simulink model "tx_to_usrp"  (R2014b)
settings: Solver=FixedStepDiscrete  SolverMode=SingleTasking  StartTime=0.0  StopTime=5  FixedStep=1/2e6  MaxStep=1/(100*40e6)  RelTol=1e-3
PreLoadFcn:
  | Fsymbol              = .5e6;         % Symbol rate
  | D=8;  % decimation / interpolation
  | Bits_per_Symbol = 2;
  | Fbit  = Bits_per_Symbol*Fsymbol;
  | 
  | FFT_Size  = 64;
  | Cyclic        = 16;
  | Pilots         = 16;
  | Pilot_Level = 8;
  | Zero_Pad  = 3;
  | QAM_Level = 6;
  | 
  | OFDM_Frame =  FFT_Size+Cyclic;
  | Symbols_per_Frame = FFT_Size-Pilots-Zero_Pad;
  | 
  | Bits_per_Frame = Bits_per_Symbol*Symbols_per_Frame;
  | 
  | F_nco = Fsymbol*D*OFDM_Frame/(Symbols_per_Frame);
  | nco_nominal=2/D;
  | 
  | 
  | Fdelay = 8;  % rrc filter delay
  | Alpha = .25;  % excess BW
  | %rrc_coef=rcosine(1,D,'fir/sqrt',Alpha,Fdelay);
  | %rrc_coef=rrc_coef/sum(rrc_coef);
  | 
  | DPS=fdesign.pulseshaping(D,'Square Root Raised Cosine','Nsym,Beta',2*Fdelay,Alpha);
  | Hd=design(DPS);
  | rrc_coef=Hd.Numerator;
  | % force DC gain to unity.
  | rrc_coef=rrc_coef/sum(rrc_coef);
  | 
  | % coefficents for Farrow filter
  | b3 = [1/6 -1/2  1/2 -1/6];
  | b2 = [1/2 -1    1/2  0];
  | b1 = [1/3  1/2 -1    1/6];
  | b0 = [0    1    0    0];
StartFcn:
  | tic
StopFcn:
  | trun=toc
undefined symbols (not defined in the file or in its folder): dfilt, j
libraries: simulink x10, dspsigops x4, dspobslib x3, commchan3 x2, commrandsrc2 x1, dspxfrm3 x1, commdigbbndam3 x1, commsdrhw_v2 x1
Description:
  | Pilot Driven OFDM  Synchronization
settings Model: Creator=Dick Benson  LastModifiedBy=lubo
settings Model: ModifiedHistory=|
  | 12/8/07  D&C
  | 12/03/08  Added BER, tuned control loops, enhanced channel model.
settings DataIOCC: SignalLoggingSaveFormat=ModelDataLogs  SaveOutput=off  SignalLogging=off  SaveTime=off  SignalLoggingName=sigsOut
settings OptimizationCC: BlockReduction=off  BooleanDataType=off  ExpressionDepthLimit=2147483647  InitFltsAndDblsToZero=on
settings DebuggingCC: SaveWithParameterizedLinksMsg=none  UnderspecifiedInitializationDetection=Classic  MergeDetectMultiDrivingBlocksExec=none  SignalResolutionControl=TryResolveAllWithWarning  SolverPrmCheckMsg=none  InheritedTsInSrcMsg=none  MultiTaskDSMMsg=warning  MultiTaskCondExecSysMsg=none  ParameterPrecisionLossMsg=none  FcnCallInpInsideContextMsg=UseLocalSettings  StateNameClashWarn=warning
settings HardwareCC: TargetUnknown=on
settings SFSimCC: SimParseCustomCode=off
settings RTWCC: IncludeERTFirstTime=on
settings GRTTargetCC: TargetFcnLib=ansi_tfl_tmw.mat  CombineOutputUpdateFcns=off  GRTInterface=on

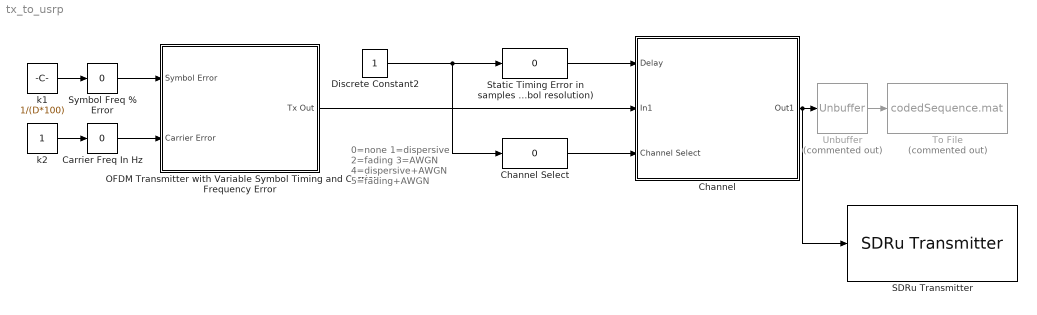
== system tx_to_usrp ==
  note: 0=none
      | 1=dispersive
      | 2=fading
      | 3=AWGN
      | 4=dispersive+AWGN
      | 5=fading+AWGN
  Carrier Freq In Hz : simulink/Math Operations/Slider Gain  low=-1000  gain=0  high=1000
  Channel : Subsystem
  Channel Select : simulink/Math Operations/Slider Gain  low=0  gain=0  high=5
  Discrete Constant2 : Constant  OutDataTypeStr=Inherit: Inherit via back propagation
  OFDM Transmitter with Variable Symbol Timing and Carrier Frequency Error : Subsystem
  SDRu Transmitter : commsdrhw_v2/SDRu Transmitter  rxtx=tx  platform=N200/N210/USRP2  USRP2_IP='192.168.10.2'  USRP_IP_X300='192.168.10.2'  USRP_IP_X310='192.168.10.2'  USRP_serialNumB200=''  USRP_serialNumB210=''  centerFrequency=8e6  centerFrequencySrc=Dialog  loOffset=0  loOffsetSrc=Dialog  masterClkRateB200=32e6  masterClkRateB210=32e6  masterClkRateX300=200e6  masterClkRateX310=200e6  masterClkRateParam=100e6  gain=8  gainSrc=Dialog  decimInterp=100  decimInterpSrc=Dialog  USRP2_IP_NUM=[49 57 50 46 49 54 56 46 49 48 46 50]  frameLength=362  outputDatatype=int16  overrunUnderrunPort=off  sampleTime=1  dboardInfo=|  HOST_DATA_PORT=30000  HOST_CONTROL_PORT=30001  USRP2_DATA_PORT=32769  USRP2_CONTROL_PORT=32768  bufferMode=Continuous streaming  EnableBurstMode=off  NumFramesInBurst=100  USRP_ID='192.168.10.2'
      | dbid: 0
      |           dbName: 'no db found'
      |          freqMin: 0
      |          freqMax: 0
      |          gainMin: 0
      |          gainMax: 0
      |     gainStepSize: 0
  Static Timing Error in samples (1/8 symbol resolution) : simulink/Math Operations/Slider Gain  low=-40  gain=0  high=40
  "Symbol Freq % Error " : simulink/Math Operations/Slider Gain  low=-0.5  gain=0  high=0.5
  To File : ToFile  Commented=on  Filename=codedSequence.mat  SaveFormat=Timeseries
  Unbuffer : Unbuffer  Commented=on  SampleBasedProcessing=Same as frame based
  k1 : Constant  Value=1/(D*100)
  k2 : Constant
  wires:
  k1/1 -> "Symbol Freq % Error "/1
  "Symbol Freq % Error "/1 -> OFDM Transmitter with Variable Symbol Timing and Carrier Frequency Error/1(Symbol Error)
  Carrier Freq In Hz/1 -> OFDM Transmitter with Variable Symbol Timing and Carrier Frequency Error/2(Carrier Error)
  k2/1 -> Carrier Freq In Hz/1
  OFDM Transmitter with Variable Symbol Timing and Carrier Frequency Error/1(Tx Out) -> Channel/2(In1)
  Discrete Constant2/1 -> Static Timing Error in samples (1/8 symbol resolution)/1, Channel Select/1
  Static Timing Error in samples (1/8 symbol resolution)/1 -> Channel/1(Delay)
  Channel Select/1 -> Channel/3(Channel Select)
  Channel/1(Out1) -> SDRu Transmitter/1, Unbuffer/1
  Unbuffer/1 -> To File/1

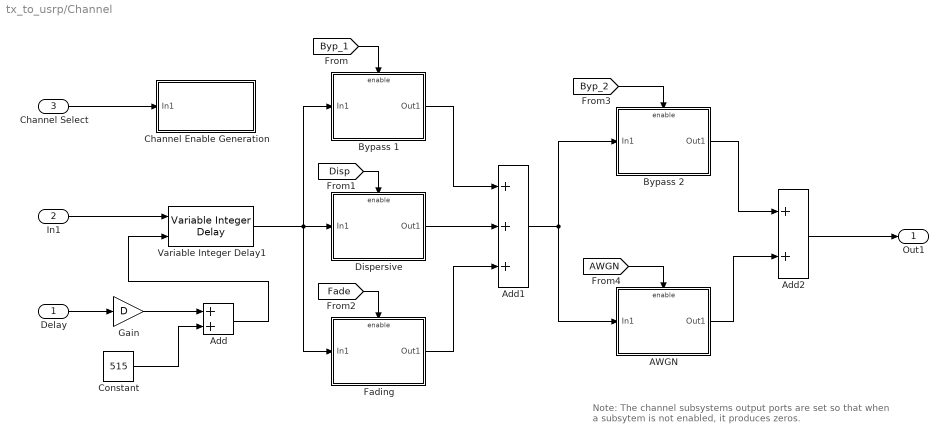
== system tx_to_usrp/Channel ==
  note: Note: The channel subsystems output ports are set so that
      | when a subsytem is not enabled, it produces zeros.
  Delay : Inport
  In1 : Inport  Port=2
  Channel Select : Inport  Port=3
  AWGN : Subsystem  TreatAsAtomicUnit=on
  Add : Sum
  Add1 : Sum  Inputs=+++
  Add2 : Sum
  Bypass 1 : Subsystem  TreatAsAtomicUnit=on
  Bypass 2 : Subsystem  TreatAsAtomicUnit=on
  Channel Enable Generation : Subsystem
  Constant : Constant  Value=515
  Dispersive : Subsystem  TreatAsAtomicUnit=on
  Fading : Subsystem  TreatAsAtomicUnit=on
  Gain : Gain  Gain=D
  Variable Integer Delay1 : dspobslib/Variable Integer Delay  dmax=2*516  InputProcessing=Columns as channels (frame based)  ic=0  noDFT=off
  Out1 : Outport
  wires:
  Delay/1 -> Gain/1
  Constant/1 -> Add/2
  Gain/1 -> Add/1
  Dispersive/1(Out1) -> Add1/2
  Bypass 1/1(Out1) -> Add1/1
  Fading/1(Out1) -> Add1/3
  Add1/1 -> AWGN/1(In1), Bypass 2/1(In1)
  Bypass 2/1(Out1) -> Add2/1
  AWGN/1(Out1) -> Add2/2
  Add2/1 -> Out1/1
  Channel Select/1 -> Channel Enable Generation/1(In1)
  [Byp_1] -> Bypass 1/Enable
  [Disp] -> Dispersive/Enable
  [Fade] -> Fading/Enable
  [Byp_2] -> Bypass 2/Enable
  [AWGN] -> AWGN/Enable
  Variable Integer Delay1/1 -> Dispersive/1(In1), Bypass 1/1(In1), Fading/1(In1)
  In1/1 -> Variable Integer Delay1/1
  Add/1 -> Variable Integer Delay1/2

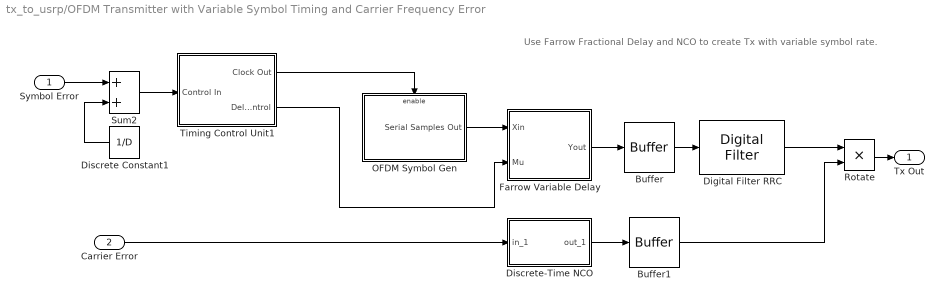
== system tx_to_usrp/OFDM Transmitter with Variable Symbol Timing and Carrier Frequency Error ==
  note: Use Farrow Fractional Delay and NCO to create Tx with variable symbol rate.
  Symbol Error : Inport
  Carrier Error : Inport  Port=2
  Buffer : Buffer  N=OFDM_Frame*D  TreatMby1Signals=One channel
  Buffer1 : Buffer  N=OFDM_Frame*D  TreatMby1Signals=One channel
  "Digital Filter RRC " : dspobslib/Digital Filter  TypePopup=FIR (all zeros)  IIRFiltStruct=Direct form II transposed  AllPoleFiltStruct=Direct form  FIRFiltStruct=Direct form  CoeffSource=Specify via dialog  NumCoeffs=rrc_coef  DenCoeffs=[1 0.1]  BiQuadCoeffs=[1 0.3 0.4 1 0.1 0.2]  LatticeCoeffs=[0.2 0.4]  denIgnore=on  FiltPerSampPopup=One filter per frame  IC=0  ICnum=0  ICden=0  roundingMode=Floor  overflowMode=off  ScaleValues=1  scaleValueFracLength=14  stageInFracLength=15  stageOutFracLength=15  FilterSource=Specify via dialog  dfiltObjectName=dfilt.dffir([1 2 1])  InputProcessing=Columns as channels (frame based)
  Discrete Constant1 : Constant  Value=1/D  OutDataTypeStr=Inherit: Inherit via back propagation
  Discrete-Time NCO : Subsystem  mask{Ac=1, Fc=0, Kc=1, Ph=0, ts=1/F_nco}
      mask prompts: Ac "Output amplitude:"; Fc "Oscillation frequency (Hz):"; Kc "Input sensitivity:"; Ph "Initial phase (rad):"; ts "Sample time:"
      mask init:
      | if ((length(Ac)~=1) | (length(Fc)~=1) | (length(Kc)~=1) | (length(Ph)~=1) | (length(ts)~=1) |(length(Ph)~=1))error('Mask parameters must be scalar values.');end;
      | pi2=2*pi;
      mask Display: disp('Discrete-Time\nNCO (rab)')
  Farrow Variable Delay : Subsystem
  OFDM Symbol Gen : Subsystem
  Rotate : Product  RndMeth=Zero
  Sum2 : Sum  SaturateOnIntegerOverflow=on  InputSameDT=on  OutDataTypeStr=Inherit: Same as first input
  Timing Control Unit1 : Subsystem
  Tx Out : Outport
  wires:
  Rotate/1 -> Tx Out/1
  Symbol Error/1 -> Sum2/1
  Farrow Variable Delay/1(Yout) -> Buffer/1
  Buffer/1 -> "Digital Filter RRC "/1
  "Digital Filter RRC "/1 -> Rotate/1
  Discrete-Time NCO/1(out_1) -> Buffer1/1
  Carrier Error/1 -> Discrete-Time NCO/1(in_1)
  Buffer1/1 -> Rotate/2
  Sum2/1 -> Timing Control Unit1/1(Control In)
  Timing Control Unit1/2(Delay Control) -> Farrow Variable Delay/2(Mu)
  Timing Control Unit1/1(Clock Out) -> OFDM Symbol Gen/Enable
  Discrete Constant1/1 -> Sum2/2
  OFDM Symbol Gen/1(Serial Samples Out) -> Farrow Variable Delay/1(Xin)

== system tx_to_usrp/Channel/AWGN ==
  In1 : Inport
  Enable : EnablePort
  AWGN Channel1 : commchan3/AWGN Channel  InputProcessing=Columns as channels (frame based)  seed=15  noiseMode="Signal to noise ratio  (SNR)"  EbNodB=10  EsNodB=10  SNRdB=15  bitsPerSym=1  Ps=1  Tsym=1  variance=1
  Out1 : Outport  OutputWhenDisabled=reset  InitialOutput=0+j*eps
  wires:
  In1/1 -> AWGN Channel1/1
  AWGN Channel1/1 -> Out1/1

== system tx_to_usrp/Channel/Bypass 1 ==
  In1 : Inport
  Enable : EnablePort
  Out1 : Outport  OutputWhenDisabled=reset  InitialOutput=0+j*eps
  wires:
  In1/1 -> Out1/1

== system tx_to_usrp/Channel/Bypass 2 ==
  In1 : Inport
  Enable : EnablePort
  Out1 : Outport  OutputWhenDisabled=reset  InitialOutput=0+j*eps
  wires:
  In1/1 -> Out1/1

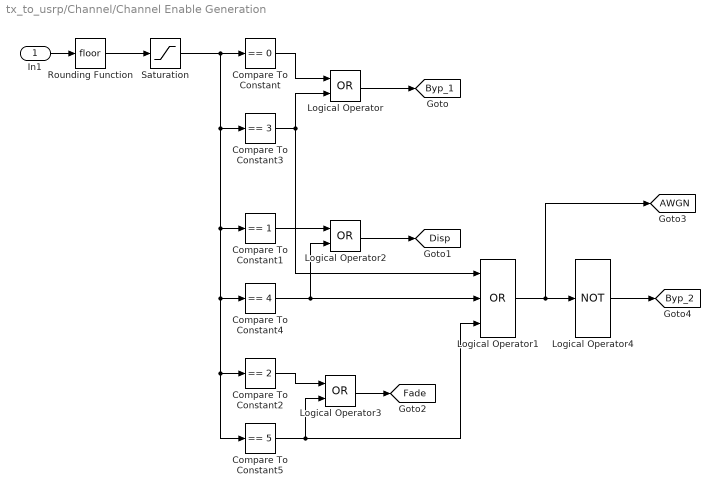
== system tx_to_usrp/Channel/Channel Enable Generation ==
  In1 : Inport
  Compare To Constant : simulink/Logic and Bit Operations/Compare To Constant  relop===  const=0  OutDataTypeStr=boolean  ZeroCross=off
  Compare To Constant1 : simulink/Logic and Bit Operations/Compare To Constant  relop===  const=1  OutDataTypeStr=boolean  ZeroCross=off
  Compare To Constant2 : simulink/Logic and Bit Operations/Compare To Constant  relop===  const=2  OutDataTypeStr=boolean  ZeroCross=off
  Compare To Constant3 : simulink/Logic and Bit Operations/Compare To Constant  relop===  const=3  OutDataTypeStr=boolean  ZeroCross=off
  Compare To Constant4 : simulink/Logic and Bit Operations/Compare To Constant  relop===  const=4  OutDataTypeStr=boolean  ZeroCross=off
  Compare To Constant5 : simulink/Logic and Bit Operations/Compare To Constant  relop===  const=5  OutDataTypeStr=boolean  ZeroCross=off
  Logical Operator : Logic  Operator=OR  AllPortsSameDT=off  OutDataTypeStr=boolean
  Logical Operator1 : Logic  Operator=OR  Inputs=3  AllPortsSameDT=off  OutDataTypeStr=boolean
  Logical Operator2 : Logic  Operator=OR  AllPortsSameDT=off  OutDataTypeStr=boolean
  Logical Operator3 : Logic  Operator=OR  AllPortsSameDT=off  OutDataTypeStr=boolean
  Logical Operator4 : Logic  Operator=NOT  Inputs=3  AllPortsSameDT=off  OutDataTypeStr=boolean
  Rounding Function : Rounding
  Saturation : Saturate  UpperLimit=5  LowerLimit=0  LinearizeAsGain=off
  tag scope: AWGN=global, Byp_1=global, Byp_2=global, Disp=global, Fade=global
  wires:
  In1/1 -> Rounding Function/1
  Compare To Constant/1 -> Logical Operator/1
  Compare To Constant3/1 -> Logical Operator/2, Logical Operator1/1
  Logical Operator/1 -> [Byp_1]
  Compare To Constant4/1 -> Logical Operator1/2, Logical Operator2/2
  Compare To Constant5/1 -> Logical Operator1/3, Logical Operator3/2
  Compare To Constant1/1 -> Logical Operator2/1
  Logical Operator2/1 -> [Disp]
  Compare To Constant2/1 -> Logical Operator3/1
  Logical Operator3/1 -> [Fade]
  Logical Operator1/1 -> Logical Operator4/1, [AWGN]
  Logical Operator4/1 -> [Byp_2]
  Rounding Function/1 -> Saturation/1
  Saturation/1 -> Compare To Constant/1, Compare To Constant1/1, Compare To Constant4/1, Compare To Constant2/1, Compare To Constant5/1, Compare To Constant3/1

== system tx_to_usrp/Channel/Dispersive ==
  In1 : Inport
  Enable : EnablePort
  Dispersive Channel : dspobslib/Digital Filter  TypePopup=FIR (all zeros)  IIRFiltStruct=Direct form II transposed  AllPoleFiltStruct=Direct form  FIRFiltStruct=Direct form  CoeffSource=Specify via dialog  NumCoeffs="[1   0  0  0.8 0 0 0 -0.7      j*.500   0 0 0 0 0 0 0  -.5  0 0 0 0 0 0 0 0 .5]/1.8"  DenCoeffs=[1 0.1]  BiQuadCoeffs=[1 0.3 0.4 1 0.1 0.2]  LatticeCoeffs=[0.2 0.4]  denIgnore=on  FiltPerSampPopup=One filter per frame  IC=0  ICnum=0  ICden=0  roundingMode=Floor  overflowMode=off  ScaleValues=1  scaleValueFracLength=14  stageInFracLength=15  stageOutFracLength=15  FilterSource=Specify via dialog  dfiltObjectName=dfilt.dffir([1 2 1])  InputProcessing=Columns as channels (frame based)
  Out1 : Outport  OutputWhenDisabled=reset  InitialOutput=0+j*eps
  wires:
  Dispersive Channel/1 -> Out1/1
  In1/1 -> Dispersive Channel/1

== system tx_to_usrp/Channel/Fading ==
  In1 : Inport
  Enable : EnablePort
  Multipath Rayleigh Fading Channel : commchan3/Multipath Rayleigh Fading Channel  maxDopplerShift=100  spectrumType=Jakes  sigmaGaussian=1/sqrt(2)  coeffRounded=[1 -1.72 0.785]  freqMinMaxRJakes=[0 1]  freqMinMaxAJakes=[0 1]  sigmaGaussian1=1/sqrt(2)  sigmaGaussian2=1/sqrt(2)  centerFreqGaussian1=0.0  centerFreqGaussian2=0.0  gainGaussian1=0.5  gainGaussian2=0.5  coeffBell=9  dopplerSpectrum=doppler.jakes  pathDelays=[0 1e-6, 3e-6]  avgPathGaindB=[0 -3, -6]  normalizePathGains=on  seed=73  enableProbe=0  openVisAtStart=off  outPathGains=off  outDelay=off
  Out1 : Outport  OutputWhenDisabled=reset  InitialOutput=0+j*eps
  wires:
  In1/1 -> Multipath Rayleigh Fading Channel/1
  Multipath Rayleigh Fading Channel/1 -> Out1/1

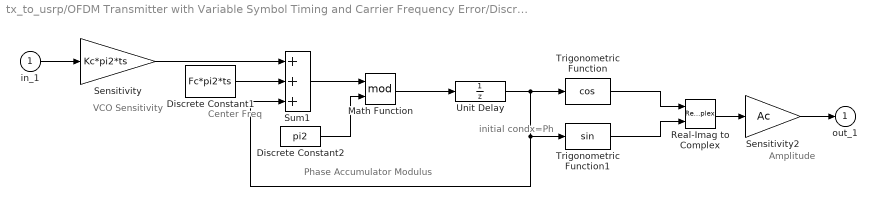
== system tx_to_usrp/OFDM Transmitter with Variable Symbol Timing and Carrier Frequency Error/Discrete-Time NCO ==
  note: initial condx=Ph
  note: VCO Sensitivity
  note: Center Freq
  note: Phase Accumulator
      | Modulus
  note: Amplitude
  in_1 : Inport
  Discrete Constant1 : Constant  Value=Fc*pi2*ts  OutDataTypeStr=Inherit: Inherit via back propagation  SampleTime=ts
  Discrete Constant2 : Constant  Value=pi2  OutDataTypeStr=Inherit: Inherit via back propagation  SampleTime=ts
  Math Function : Math  Operator=mod  SaturateOnIntegerOverflow=on
  Real-Imag to Complex : RealImagToComplex
  Sensitivity : Gain  Gain=Kc*pi2*ts  SaturateOnIntegerOverflow=on  OutDataTypeStr=Inherit: Same as input  ParamDataTypeStr=Inherit: Same as input
  Sensitivity2 : Gain  Gain=Ac  SaturateOnIntegerOverflow=on  OutDataTypeStr=Inherit: Same as input  ParamDataTypeStr=Inherit: Same as input
  Sum1 : Sum  Inputs=+++  SaturateOnIntegerOverflow=on  InputSameDT=on  OutDataTypeStr=Inherit: Same as first input
  Trigonometric Function : Trigonometry  Operator=cos
  Trigonometric Function1 : Trigonometry
  Unit Delay : UnitDelay  InitialCondition=Ph  SampleTime=ts
  out_1 : Outport
  wires:
  Real-Imag to Complex/1 -> Sensitivity2/1
  Trigonometric Function1/1 -> Real-Imag to Complex/2
  Discrete Constant2/1 -> Math Function/2
  Sum1/1 -> Math Function/1
  Math Function/1 -> Unit Delay/1
  in_1/1 -> Sensitivity/1
  Sensitivity/1 -> Sum1/1
  Unit Delay/1 -> Trigonometric Function/1, Trigonometric Function1/1, Sum1/3
  Trigonometric Function/1 -> Real-Imag to Complex/1
  Sensitivity2/1 -> out_1/1
  Discrete Constant1/1 -> Sum1/2

== system tx_to_usrp/OFDM Transmitter with Variable Symbol Timing and Carrier Frequency Error/Farrow Variable Delay ==
  Xin : Inport
  Mu : Inport  Port=2
  Filter State : Subsystem
  MADS : Subsystem
  Yout : Outport
  wires:
  Filter State/1(Out1) -> MADS/1(In1)
  Xin/1 -> Filter State/1(In1)
  Mu/1 -> MADS/2(mu)
  MADS/1(Yout) -> Yout/1

== system tx_to_usrp/OFDM Transmitter with Variable Symbol Timing and Carrier Frequency Error/OFDM Symbol Gen ==
  note: Output Samples Serially
  note: Note: Ouptut is SET TO ZERO
      | when not enabled.
      | This effecitvly inserts ZEROS in the stream
      | for proper interpolation.
  Enable : EnablePort
  Divide by OFDM_Frame length : Subsystem  TreatAsAtomicUnit=on  mask(Pulse Divider){div=OFDM_Frame, ph=0}
      mask prompts: div "Modulo:"; ph "Initial Phase Delay (cycles):"
  OFDM Generator : Subsystem
  Selector : Selector  InputPortWidth=80  IndexOptions=Index vector (port)  Indices=[1 3]
  Serial Samples Out : Outport  OutputWhenDisabled=reset  InitialOutput=0+j*eps
  wires:
  OFDM Generator/1(Out1) -> Selector/1
  Divide by OFDM_Frame length/1(Enable) -> OFDM Generator/Enable
  Selector/1 -> Serial Samples Out/1
  Divide by OFDM_Frame length/2(Count) -> Selector/2

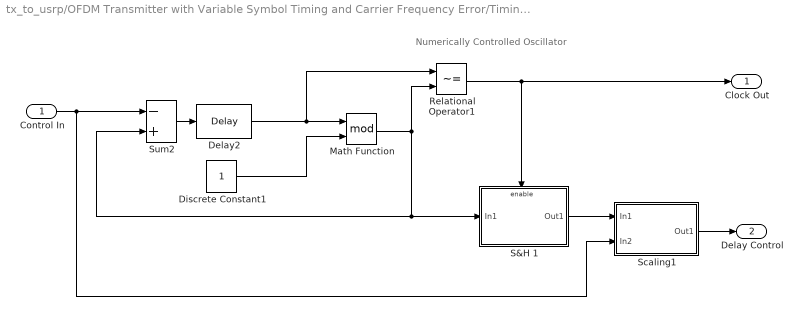
== system tx_to_usrp/OFDM Transmitter with Variable Symbol Timing and Carrier Frequency Error/Timing Control Unit1 ==
  note: Numerically Controlled Oscillator
  Control In : Inport
  Delay2 : dspsigops/Delay  dly_unit=Samples  delay=1  ic_detail=on  dif_ic_for_ch=off  dif_ic_for_dly=off  ic=0  reset_popup=None
  Discrete Constant1 : Constant  OutDataTypeStr=Inherit: Inherit via back propagation
  Math Function : Math  Operator=mod  SaturateOnIntegerOverflow=on
  Relational Operator1 : RelationalOperator  Operator=~=  OutDataTypeStr=boolean
  S&H 1 : Subsystem  TreatAsAtomicUnit=on
  Scaling1 : Subsystem
  Sum2 : Sum  Inputs=-+  SaturateOnIntegerOverflow=on  InputSameDT=on  OutDataTypeStr=Inherit: Same as first input
  Clock Out : Outport
  Delay Control : Outport  Port=2
  wires:
  Scaling1/1(Out1) -> Delay Control/1
  S&H 1/1(Out1) -> Scaling1/1(In1)
  Delay2/1 -> Math Function/1, Relational Operator1/1
  Discrete Constant1/1 -> Math Function/2
  Sum2/1 -> Delay2/1
  Math Function/1 -> Relational Operator1/2, S&H 1/1(In1), Sum2/2
  Relational Operator1/1 -> Clock Out/1, S&H 1/Enable
  Control In/1 -> Sum2/1, Scaling1/2(In2)

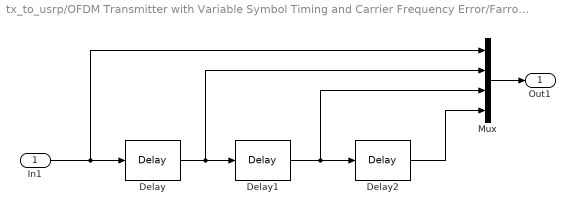
== system tx_to_usrp/OFDM Transmitter with Variable Symbol Timing and Carrier Frequency Error/Farrow Variable Delay/Filter State ==
  In1 : Inport
  Delay : dspsigops/Delay  dly_unit=Samples  delay=1  ic_detail=off  dif_ic_for_ch=off  dif_ic_for_dly=off  ic=0  reset_popup=None
  Delay1 : dspsigops/Delay  dly_unit=Samples  delay=1  ic_detail=off  dif_ic_for_ch=off  dif_ic_for_dly=off  ic=0  reset_popup=None
  Delay2 : dspsigops/Delay  dly_unit=Samples  delay=1  ic_detail=off  dif_ic_for_ch=off  dif_ic_for_dly=off  ic=0  reset_popup=None
  Mux : Mux
  Out1 : Outport
  wires:
  In1/1 -> Delay/1, Mux/1
  Delay/1 -> Mux/2, Delay1/1
  Delay1/1 -> Mux/3, Delay2/1
  Delay2/1 -> Mux/4
  Mux/1 -> Out1/1

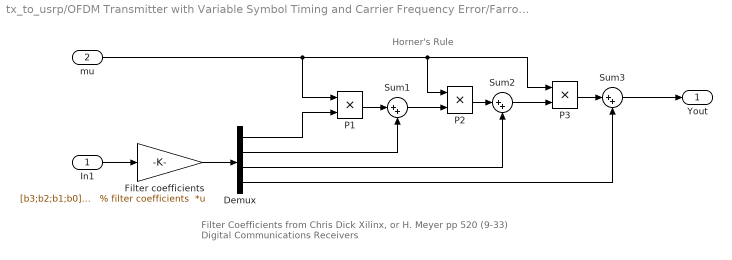
== system tx_to_usrp/OFDM Transmitter with Variable Symbol Timing and Carrier Frequency Error/Farrow Variable Delay/MADS ==
  note: Horner's Rule
  note: Filter Coefficients from Chris Dick Xilinx,
      | or H. Meyer pp 520 (9-33) Digital Communications Receivers
  In1 : Inport
  mu : Inport  Port=2
  Demux : Demux
  Filter coefficients : Gain  Gain="[b3;b2;b1;b0]   % filter coefficients"  Multiplication=Matrix(K*u)  SaturateOnIntegerOverflow=on  OutDataTypeStr=Inherit: Same as input  ParamDataTypeStr=Inherit: Same as input
  P1 : Product  SaturateOnIntegerOverflow=on  OutDataTypeStr=Inherit: Same as first input
  P2 : Product  SaturateOnIntegerOverflow=on  OutDataTypeStr=Inherit: Same as first input
  P3 : Product  SaturateOnIntegerOverflow=on  OutDataTypeStr=Inherit: Same as first input
  Sum1 : Sum  Inputs=|++  SaturateOnIntegerOverflow=on
  Sum2 : Sum  Inputs=|++  SaturateOnIntegerOverflow=on
  Sum3 : Sum  Inputs=|++  SaturateOnIntegerOverflow=on
  Yout : Outport
  wires:
  P3/1 -> Sum3/1
  P2/1 -> Sum2/1
  Filter coefficients/1 -> Demux/1
  In1/1 -> Filter coefficients/1
  mu/1 -> P3/1, P2/1, P1/1
  Demux/1 -> P1/2
  Sum1/1 -> P2/2
  Sum2/1 -> P3/2
  Demux/2 -> Sum1/2
  P1/1 -> Sum1/1
  Demux/3 -> Sum2/2
  Demux/4 -> Sum3/2
  Sum3/1 -> Yout/1

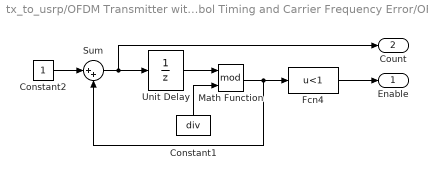
== system tx_to_usrp/OFDM Transmitter with Variable Symbol Timing and Carrier Frequency Error/OFDM Symbol Gen/Divide by OFDM_Frame length ==
  Constant1 : Constant  Value=div
  Constant2 : Constant
  Fcn4 : Fcn  Expr=u<1
  Math Function : Math  Operator=mod  SaturateOnIntegerOverflow=on
  Sum : Sum  Inputs=|++  SaturateOnIntegerOverflow=on  InputSameDT=on  OutDataTypeStr=Inherit: Same as first input
  Unit Delay : UnitDelay  InitialCondition=div-ph  SampleTime=-1
  Enable : Outport
  Count : Outport  Port=2
  wires:
  Sum/1 -> Unit Delay/1, Count/1
  Constant2/1 -> Sum/1
  Unit Delay/1 -> Math Function/1
  Math Function/1 -> Sum/2, Fcn4/1
  Constant1/1 -> Math Function/2
  Fcn4/1 -> Enable/1

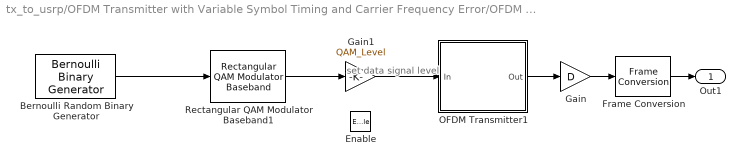
== system tx_to_usrp/OFDM Transmitter with Variable Symbol Timing and Carrier Frequency Error/OFDM Symbol Gen/OFDM Generator ==
  note: set data signal level
  Enable : EnablePort
  Bernoulli Random Binary Generator : commrandsrc2/Bernoulli Binary Generator  P=0.5  seed=123  Ts=-1  frameBased=on  sampPerFrame=Bits_per_Frame  orient=off  outDataType=double
  Frame Conversion : FrameConversion  OutFrame=Sample-based
  Gain : Gain  Gain=D
  Gain1 : Gain  Gain=QAM_Level  SaturateOnIntegerOverflow=on  OutDataTypeStr=Inherit: Same as input  ParamDataTypeStr=Inherit: Same as input
  OFDM Transmitter1 : Subsystem
      mask Display: disp('OFDM\nTransmitter')
  Rectangular QAM Modulator Baseband1 : commdigbbndam3/Rectangular QAM Modulator Baseband  M=4  InType=Bit  Enc=Binary  Mapping=[0:15]  PowType=Min. distance between symbols  MinDist=2  AvgPow=1  PeakPow=1  Ph=0  outDtype=double  outWordLen=16  outUDDataType=sfix(16)  outFracLenMode=Best precision  outFracLen=15
  Out1 : Outport
  wires:
  Bernoulli Random Binary Generator/1 -> Rectangular QAM Modulator Baseband1/1
  OFDM Transmitter1/1(Out) -> Gain/1
  Rectangular QAM Modulator Baseband1/1 -> Gain1/1
  Gain/1 -> Frame Conversion/1
  Gain1/1 -> OFDM Transmitter1/1(In)
  Frame Conversion/1 -> Out1/1

== system tx_to_usrp/OFDM Transmitter with Variable Symbol Timing and Carrier Frequency Error/Timing Control Unit1/S&H 1 ==
  In1 : Inport
  Enable : EnablePort
  Out1 : Outport
  wires:
  In1/1 -> Out1/1

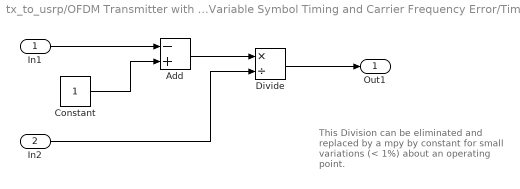
== system tx_to_usrp/OFDM Transmitter with Variable Symbol Timing and Carrier Frequency Error/Timing Control Unit1/Scaling1 ==
  note: This Division can be eliminated
      | and replaced by a mpy by constant
      | for small variations (< 1%)
      | about an operating point.
  In1 : Inport
  In2 : Inport  Port=2
  Add : Sum  Inputs=-+
  Constant : Constant
  Divide : Product  Inputs=*/
  Out1 : Outport
  wires:
  In2/1 -> Divide/2
  In1/1 -> Add/1
  Constant/1 -> Add/2
  Add/1 -> Divide/1
  Divide/1 -> Out1/1

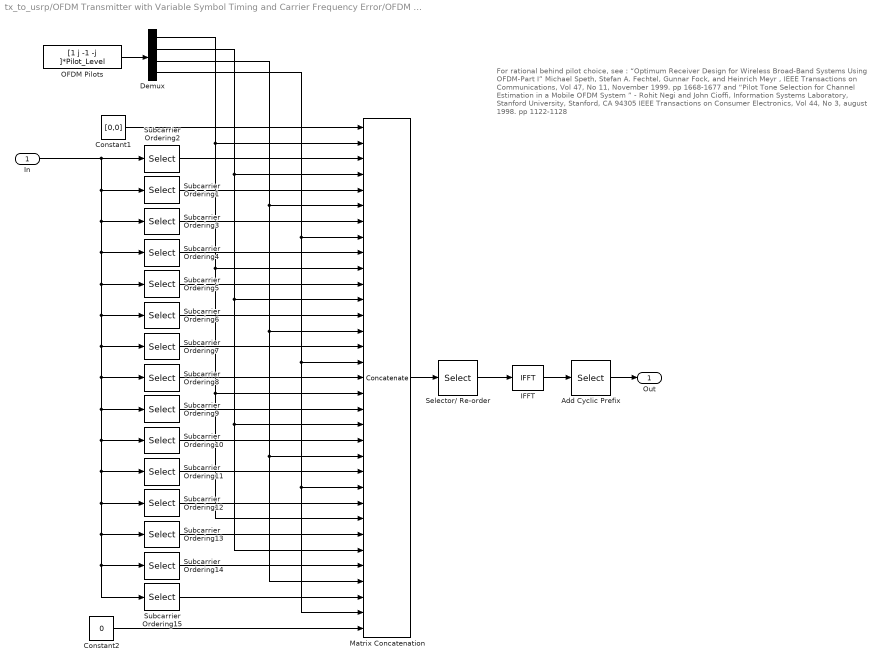
== system tx_to_usrp/OFDM Transmitter with Variable Symbol Timing and Carrier Frequency Error/OFDM Symbol Gen/OFDM Generator/OFDM Transmitter1 ==
  note: For rational behind pilot choice, see :
      | “Optimum Receiver Design for Wireless Broad-Band Systems Using OFDM-Part I”
      | Michael Speth, Stefan A. Fechtel, Gunnar Fock, and Heinrich Meyr ,
      |  IEEE Transactions on Communications, Vol 47, No 11, November 1999. pp 1668-1677
      | and
      | “Pilot Tone Selection for Channel Estimation in a Mobile OFDM System ” -
      |  Rohit Negi and John Cioffi, Information Systems Laboratory, Stanford University, Stanford, CA 94305
      | IEEE Transactions on Consumer Electronics, Vol 44, No 3, august 1998. pp 1122-1128
  In : Inport
  Add Cyclic Prefix : Selector  InputPortWidth=64  Indices=[49:64 1:64]
  Constant1 : Constant  Value=[0,0]
  Constant2 : Constant  Value=0
  Demux : Demux
  IFFT : dspxfrm3/IFFT  CompMethod=Table lookup  TableOpt=HYBRID  TableOptActive=Speed  BitRevOrder=off  cs_in=off  SkipNorm=on  InheritFFTLength=on  FFTLength=64  WrapInput=on  mode=Complex  outSamplingMode=Frame based  RowConvenienceOn=on  FFTImplementation=Auto  firstCoeffDataTypeStr=Inherit: Same word length as input  firstCoeffLastDataTypeStr=Inherit: Same word length as input  outputMin=[]  outputMax=[]  roundingMode=Floor  overflowMode=off
  Matrix Concatenation : Concatenate  NumInputs=33  Mode=Multidimensional array
  OFDM Pilots : Constant  Value="[1 j -1 -j   ]*Pilot_Level"
  Selector/ Re-order : Selector  InputPortWidth=64  Indices=[33:64 1:32]
  Subcarrier Ordering1 : Selector  InputPortWidth=Symbols_per_Frame  Indices=4:6
  Subcarrier Ordering10 : Selector  InputPortWidth=Symbols_per_Frame  Indices=28:30
  Subcarrier Ordering11 : Selector  InputPortWidth=Symbols_per_Frame  Indices=31:33
  Subcarrier Ordering12 : Selector  InputPortWidth=Symbols_per_Frame  Indices=34:36
  Subcarrier Ordering13 : Selector  InputPortWidth=Symbols_per_Frame  Indices=37:39
  Subcarrier Ordering14 : Selector  InputPortWidth=Symbols_per_Frame  Indices=40:42
  Subcarrier Ordering15 : Selector  InputPortWidth=Symbols_per_Frame  Indices=43:45
  Subcarrier Ordering2 : Selector  InputPortWidth=Symbols_per_Frame  Indices=1:3
  Subcarrier Ordering3 : Selector  InputPortWidth=Symbols_per_Frame  Indices=7:9
  Subcarrier Ordering4 : Selector  InputPortWidth=Symbols_per_Frame  Indices=10:12
  Subcarrier Ordering5 : Selector  InputPortWidth=Symbols_per_Frame  Indices=13:15
  Subcarrier Ordering6 : Selector  InputPortWidth=Symbols_per_Frame  Indices=16:18
  Subcarrier Ordering7 : Selector  InputPortWidth=Symbols_per_Frame  Indices=19:21
  Subcarrier Ordering8 : Selector  InputPortWidth=Symbols_per_Frame  Indices=22:24
  Subcarrier Ordering9 : Selector  InputPortWidth=Symbols_per_Frame  Indices=25:27
  Out : Outport
  wires:
  In/1 -> Subcarrier Ordering14/1, Subcarrier Ordering15/1, Subcarrier Ordering13/1, Subcarrier Ordering12/1, Subcarrier Ordering11/1, Subcarrier Ordering10/1, Subcarrier Ordering9/1, Subcarrier Ordering8/1, Subcarrier Ordering7/1, Subcarrier Ordering6/1, Subcarrier Ordering5/1, Subcarrier Ordering4/1, Subcarrier Ordering3/1, Subcarrier Ordering1/1, Subcarrier Ordering2/1
  IFFT/1 -> Add Cyclic Prefix/1
  Matrix Concatenation/1 -> Selector/ Re-order/1
  Selector/ Re-order/1 -> IFFT/1
  Subcarrier Ordering2/1 -> Matrix Concatenation/3
  Subcarrier Ordering1/1 -> Matrix Concatenation/5
  Subcarrier Ordering3/1 -> Matrix Concatenation/7
  Subcarrier Ordering4/1 -> Matrix Concatenation/9
  Subcarrier Ordering5/1 -> Matrix Concatenation/11
  Subcarrier Ordering6/1 -> Matrix Concatenation/13
  Subcarrier Ordering7/1 -> Matrix Concatenation/15
  Subcarrier Ordering8/1 -> Matrix Concatenation/17
  Subcarrier Ordering9/1 -> Matrix Concatenation/19
  Subcarrier Ordering10/1 -> Matrix Concatenation/21
  Subcarrier Ordering11/1 -> Matrix Concatenation/23
  Subcarrier Ordering12/1 -> Matrix Concatenation/25
  Subcarrier Ordering13/1 -> Matrix Concatenation/27
  Subcarrier Ordering14/1 -> Matrix Concatenation/29
  Subcarrier Ordering15/1 -> Matrix Concatenation/31
  Add Cyclic Prefix/1 -> Out/1
  Constant1/1 -> Matrix Concatenation/1
  Constant2/1 -> Matrix Concatenation/33
  Demux/2 -> Matrix Concatenation/4, Matrix Concatenation/12, Matrix Concatenation/20, Matrix Concatenation/28
  Demux/3 -> Matrix Concatenation/6, Matrix Concatenation/14, Matrix Concatenation/22, Matrix Concatenation/30
  Demux/4 -> Matrix Concatenation/8, Matrix Concatenation/16, Matrix Concatenation/24, Matrix Concatenation/32
  OFDM Pilots/1 -> Demux/1
  Demux/1 -> Matrix Concatenation/26, Matrix Concatenation/18, Matrix Concatenation/10, Matrix Concatenation/2
